simulink model "pe_estimation_centre"  (Simulink 8.7)
settings: Solver=FixedStepDiscrete  SolverMode=SingleTasking  StartTime=0.0  StopTime=5000e-3  FixedStep=1/100000  RelTol=1e-3  AbsTol=1e-6
libraries: commchan3 x1, commsink2 x1, dspsrcs4 x1
settings Model: Creator=amoura  LastModifiedBy=Artur Moura
settings DataIOCC: LimitDataPoints=off  SignalLoggingSaveFormat=ModelDataLogs  SignalLoggingName=sigsOut
settings OptimizationCC: BooleanDataType=off  ExpressionDepthLimit=2147483647  InitFltsAndDblsToZero=on
settings DebuggingCC: SaveWithParameterizedLinksMsg=none  SignalResolutionControl=TryResolveAllWithWarning  MultiTaskDSMMsg=warning  MultiTaskCondExecSysMsg=none  FcnCallInpInsideContextMsg=UseLocalSettings  StateNameClashWarn=warning
settings HardwareCC: TargetUnknown=on
settings RTWCC: TemplateMakefile=grt_unix.tmf
settings GRTTargetCC: TargetFcnLib=ansi_tfl_tmw.mat  ModelReferenceCompliant=off  CombineOutputUpdateFcns=off  MatFileLogging=off  GRTInterface=on

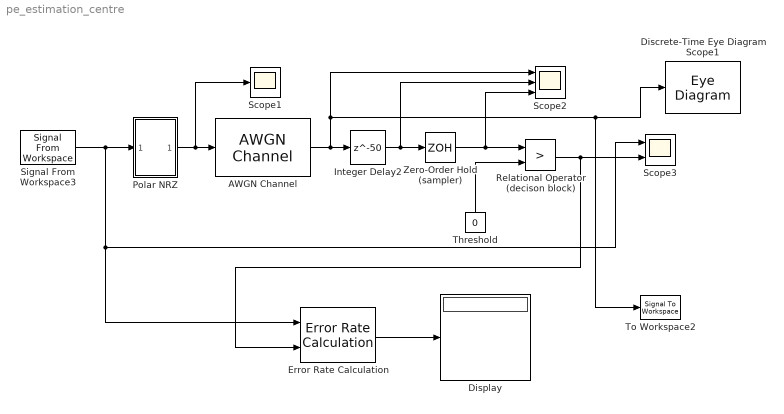
== system pe_estimation_centre ==
  AWGN Channel : commchan3/AWGN Channel  InputProcessing=Columns as channels (frame based)  seed=53  noiseMode=Variance from mask  EbNodB=10  EsNodB=10  SNRdB=10  bitsPerSym=1  Ps=1  Tsym=1  variance=0.2
  Discrete-Time Eye Diagram Scope1 : EyeDiagram  Tag=EyeDiagram
  Display : Display
  Error Rate Calculation : commsink2/Error Rate Calculation  N=1  st_delay=0  cp_mode=Entire frame  subframe=[]  PMode=Port  WsName=ErrorVec  RsMode2=off  stop=off  numErr=100  maxBits=1e6
  Integer Delay2 : Delay  DelayLength=50  InputProcessing=Inherited  SampleTime=1/100000
  Polar NRZ : Subsystem  mask(Polar NRZ){}
      mask help:
      | This block encodes a unipolar NRZ signal into the polar NRZ line code
      |
      | The output values are +1 for a nonzero input and -1 for a zero one.
      mask Display: disp('Polar\nNRZ')
  Relational Operator (decison block) : RelationalOperator  Operator=>  InputSameDT=on
  Scope1 : Scope
  Scope2 : Scope  NumInputPorts=3
  Scope3 : Scope  NumInputPorts=2
  Signal From Workspace3 : dspsrcs4/Signal From Workspace  X=randi([0 1],10000,1)  Ts=1/1000  nsamps=1  OutputAfterFinalValue=Cyclic repetition  ignoreOrWarnInputAndFrameLengths=off  OutputFrames=on
  Threshold : Constant  Value=0
  To Workspace2 : SignalToWorkspace  VariableName=simout
  Zero-Order Hold (sampler) : ZeroOrderHold  SampleTime=1/1000
  wires:
  Relational Operator (decison block)/1 -> Error Rate Calculation/2, Scope3/2
  Zero-Order Hold (sampler)/1 -> Relational Operator (decison block)/1, Scope2/3
  Polar NRZ/1(Out1) -> Scope1/1, AWGN Channel/1
  Signal From Workspace3/1 -> Polar NRZ/1(In1), Error Rate Calculation/1, Scope3/1
  Error Rate Calculation/1 -> Display/1
  Threshold/1 -> Relational Operator (decison block)/2
  AWGN Channel/1 -> Discrete-Time Eye Diagram Scope1/1, To Workspace2/1, Scope2/1, Integer Delay2/1
  Integer Delay2/1 -> Zero-Order Hold (sampler)/1, Scope2/2

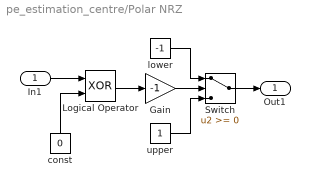
== system pe_estimation_centre/Polar NRZ ==
  In1 : Inport
  Gain : Gain  Gain=-1  SaturateOnIntegerOverflow=on  OutDataTypeStr=Inherit: Same as input  ParamDataTypeStr=Inherit: Same as input
  Logical Operator : Logic  Operator=XOR
  Switch : Switch  SaturateOnIntegerOverflow=on  InputSameDT=on
  const : Constant  Value=0
  lower : Constant  Value=-1
  upper : Constant
  Out1 : Outport
  wires:
  In1/1 -> Logical Operator/1
  lower/1 -> Switch/1
  upper/1 -> Switch/3
  Gain/1 -> Switch/2
  Switch/1 -> Out1/1
  Logical Operator/1 -> Gain/1
  const/1 -> Logical Operator/2
